simulink model "temp_bangbang"  (R2018a)
settings: Solver=FixedStepAuto  StartTime=0.0  StopTime=20000  FixedStep=1  RelTol=1e-3
undefined symbols (not defined in the file): daq
libraries: daqlib x3
settings Model: Creator=matthew  LastModifiedBy=matthew

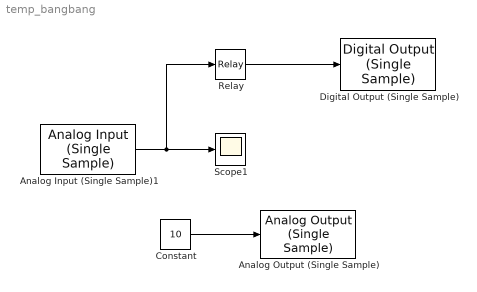
== system temp_bangbang ==
  Analog Input (Single Sample)1 : daqlib/Analog Input (Single Sample)  DeviceMenu=ni myDAQ1 (NI myDAQ)  Device=ni myDAQ1 (NI myDAQ)  ObjConstructor=daq.createSession('ni')  BlockSampleTime=1  NChannelsSelected=1  Channels=1$ai0$$myDAQ1$1$2$1$1$#0$ai1$$myDAQ1$1$1$1$1$#  NPorts=1 for all channels  OutputTimestamp=off
      settings: SourceProductName=Data Acquisition Toolbox  SourceProductBaseCode=DA
  Analog Output (Single Sample) : daqlib/Analog Output (Single Sample)  DeviceMenu=ni myDAQ1 (NI myDAQ)  Device=ni myDAQ1 (NI myDAQ)  ObjConstructor=daq.createSession('ni')  NChannelsSelected=1  Channels=1$ao0$$myDAQ1$1$2$N/A$#0$ao1$$myDAQ1$1$2$N/A$#  NPorts=1 for all channels  BlockSampleTime=1
      settings: SourceProductName=Data Acquisition Toolbox  SourceProductBaseCode=DA
  Constant : Constant  Value=10
  Digital Output (Single Sample) : daqlib/Digital Output (Single Sample)  DeviceMenu=ni myDAQ1 (NI myDAQ)  Device=ni myDAQ1 (NI myDAQ)  ObjConstructor=daq.createSession('ni')  BlockSampleTime=1  IsDigitalInput=off  NLinesSelected=1  Lines=1$port0/line0$$myDAQ1$#0$port0/line1$$myDAQ1$#0$port0/line2$$myDAQ1$#0$port0/line3$$myDAQ1$#0$port0/line4$$myDAQ1$#0$port0/line5$$myDAQ1$#0$port0/line6$$myDAQ1$#0$port0/line7$$myDAQ1$#  NPorts=1 for all lines
      settings: SourceProductName=Data Acquisition Toolbox  SourceProductBaseCode=DA
  Relay : Relay  OnSwitchValue=4.61  OffSwitchValue=4.6  OutDataTypeStr=boolean
  Scope1 : Scope
  wires:
  Analog Input (Single Sample)1/1 -> Relay/1, Scope1/1
  Relay/1 -> Digital Output (Single Sample)/1
  Constant/1 -> Analog Output (Single Sample)/1
